simulink model "FB_M"  (Simulink 8.6)
settings: Solver=VariableStepAuto  StartTime=0.0  StopTime=50  RelTol=1e-3
values from neighbouring files (symbols this model uses):
  bHI = 0    [Initiation.m]
  m = 1    [Initiation.m]
  nWall = block.DialogPrm(6).Data    [Controller1.m]    (also in HapticController.m = block.DialogPrm(3).Data; Initial_Conditions.m = -1; Initiation.m = -1; MoreConservative.m = block.DialogPrm(5).Data)
  tsampling = block.DialogPrm(3).Data    [Controller.m]    (also in Controller1.m; Controller_more.m = block.DialogPrm(4).Data; HapticController.m = block.DialogPrm(6).Data; Initial_Conditions.m = 0.001)
  x0 = block.DialogPrm(5).Data    [HapticDevice.m]    (also in HumanOperator.m; LessConservative.m = block.DialogPrm(3).Data; MoreConservative.m = block.DialogPrm(3).Data)
  xWall = 0.126    [Initiation.m]    (also in MoreConservative.m = block.DialogPrm(4).Data; Parameters.m = [1 2 3 4 5 6 7 8]*0.0005; VirtualEnvironment.m = block.DialogPrm(3).Data; VirtualEnvironment5.m = block.DialogPrm(4).Data)
undefined symbols (not defined in the file or in its folder): x_dot0
settings Model: Creator=TOSHIBA  LastModifiedBy=TOSHIBA
settings DataIOCC: SaveFormat=Dataset  SignalLoggingSaveFormat=Dataset
settings OptimizationCC: ExpressionDepthLimit=128
settings DebuggingCC: UnderspecifiedInitializationDetection=Simplified  MergeDetectMultiDrivingBlocksExec=error  SolverPrmCheckMsg=none  FcnCallInpInsideContextMsg=EnableAllAsError  StateNameClashWarn=none
settings HardwareCC: ProdBitPerPointer=64  ProdLargestAtomicFloat=Float  ProdIntDivRoundTo=Zero  ProdEndianess=LittleEndian  ProdWordSize=64  ProdHWDeviceType=Intel->x86-64 (Windows64)
settings GRTTargetCC: GeneratePreprocessorConditionals=Use local settings  CombineOutputUpdateFcns=on  GRTInterface=off
settings ConfigComp: CovModelRefEnable=off

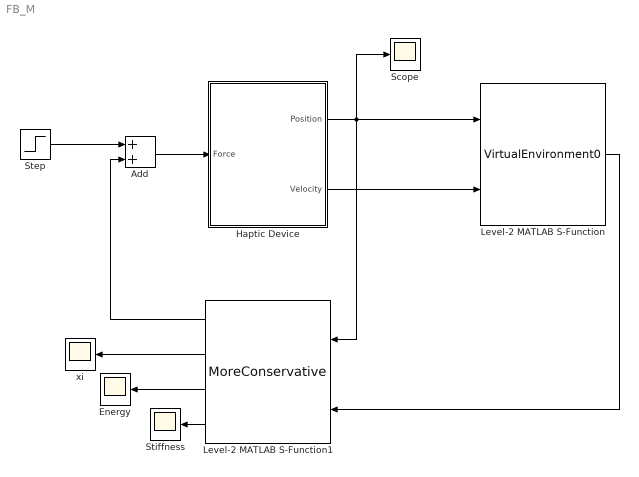
== system FB_M ==
  Add : Sum
  Energy : Scope
  Haptic Device : Subsystem
  Level-2 MATLAB S-Function : M-S-Function  FunctionName=VirtualEnvironment0  Parameters=kWall, bWall, nWall, xWall, tsampling
  Level-2 MATLAB S-Function1 : M-S-Function  FunctionName=MoreConservative  Parameters=0.1*bHI, tsampling, x0, xWall, nWall
  Scope : Scope
  Step : Step  Time=0.35  After=-10  SampleTime=0
  Stiffness : Scope
  xi : Scope
  wires:
  Add/1 -> Haptic Device/1(Force)
  Haptic Device/1(Position) -> Level-2 MATLAB S-Function1/1, Level-2 MATLAB S-Function/1, Scope/1
  Step/1 -> Add/1
  Level-2 MATLAB S-Function1/1 -> Add/2
  Level-2 MATLAB S-Function/1 -> Level-2 MATLAB S-Function1/2
  Haptic Device/2(Velocity) -> Level-2 MATLAB S-Function/2
  Level-2 MATLAB S-Function1/4 -> Stiffness/1
  Level-2 MATLAB S-Function1/3 -> Energy/1
  Level-2 MATLAB S-Function1/2 -> xi/1

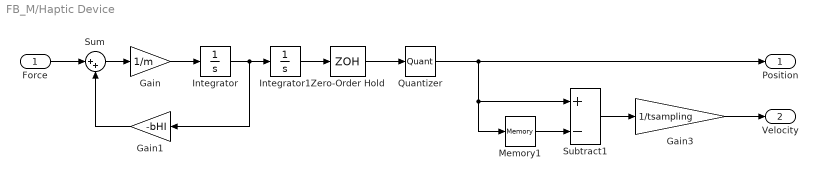
== system FB_M/Haptic Device ==
  Force : Inport
  Gain : Gain  Gain=1/m
  Gain1 : Gain  Gain=-bHI
  Gain3 : Gain  Gain=1/tsampling
  Integrator : Integrator  InitialCondition=x_dot0
  Integrator1 : Integrator  InitialCondition=x0
  Memory1 : Memory  X0=x0
  Quantizer : Quantizer  QuantizationInterval=0.00002
  Subtract1 : Sum  Inputs=+-
  Sum : Sum  Inputs=|++
  Zero-Order Hold : ZeroOrderHold  SampleTime=tsampling
  Position : Outport
  Velocity : Outport  Port=2
  wires:
  Integrator1/1 -> Zero-Order Hold/1
  Gain/1 -> Integrator/1
  Sum/1 -> Gain/1
  Gain1/1 -> Sum/2
  Integrator/1 -> Gain1/1, Integrator1/1
  Force/1 -> Sum/1
  Subtract1/1 -> Gain3/1
  Memory1/1 -> Subtract1/2
  Gain3/1 -> Velocity/1
  Zero-Order Hold/1 -> Quantizer/1
  Quantizer/1 -> Memory1/1, Subtract1/1, Position/1
